simulink model "Aufgabe1_Bremsvorgang"  (R2022b)
settings: Solver=VariableStepAuto  StartTime=0.0  StopTime=10.0  RelTol=1e-3
undefined symbols (not defined in the file or in its folder): s
settings Model: Creator=tinah  LastModifiedBy=tinah

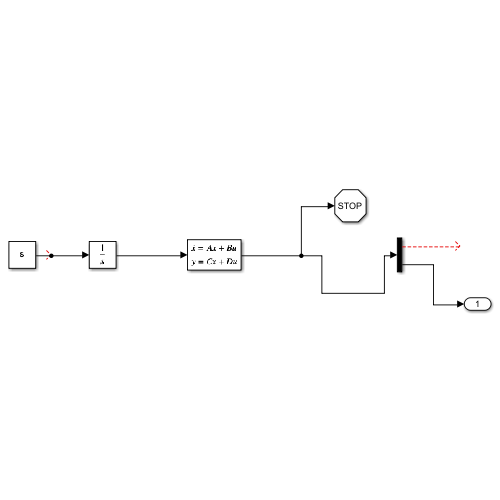
[thumbnail: Simulink's stored preview of the top-level diagram]
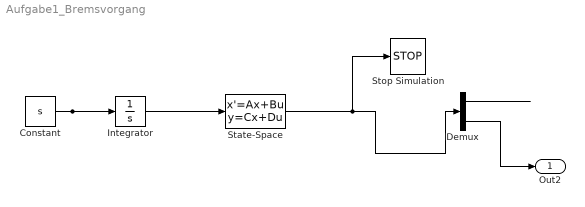
== system Aufgabe1_Bremsvorgang ==
  Constant : Constant  Value=s
  Demux : Demux  Outputs=2
  Integrator : Integrator
  State-Space : StateSpace  A=[0 1; 0 0]  B=[0; 1]  C=[1 0; 0 1]  D=[0;0]  InitialCondition=0
  Stop Simulation : Stop
  Out2 : Outport
  wires:
  Demux/1 -> ?
  Demux/2 -> Out2/1
  State-Space/1 -> Demux/1, Stop Simulation/1
  Constant/1 -> Integrator/1
  Integrator/1 -> State-Space/1
